simulink model "district_heating"  (R2018b)
settings: Solver=VariableStepAuto  StartTime=0.0  StopTime=24*3600  RelTol=1e-3
undefined symbols (not defined in the file): path_carnot
libraries: carnot x16, Pipe_BiFlow x2
settings Model: Creator=drhf  LastModifiedBy=drhf
settings SolverCC: AlgebraicLoopSolver=LineSearch

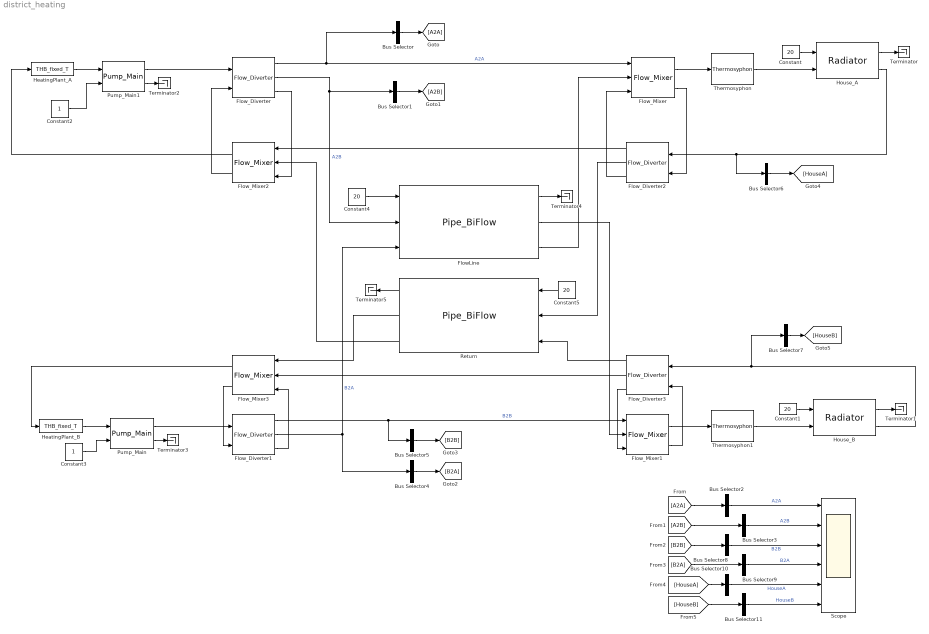
== system district_heating ==
  Bus Selector{,1,4..7} (6 alike) : BusSelector  OutputSignals=Temperature,MassFlow  OutputAsBus=on
  Bus Selector{2..3,8..11} (6 alike) : BusSelector  OutputSignals=MassFlow  OutputAsBus=on
  Constant{,1,4..5} (4 alike) : Constant  Value=20
  Constant2 : Constant
  Constant3 : Constant
  FlowLine : Pipe_BiFlow/Pipe_BiFlow  t0=20  hgt=254.6479  stgtype=1  tini=[20 20 20 20 20 20 20 20 20 20]  mpts=[1 2 3 4 5 6 7 8 9 10]  PathName=fullfile(path_carnot('libsl'),'Storage','Thermal','Storage_Type_1','parameter_set')  FileName='<user defined>'  userPath=off  userParam=on  uwall=1  ubot=1  utop=1  axcond=1  volume=2  dia=0.1  standing=standing cylinder  nodes=10  mpoints=10  pipe1inlet=1  pipe1outlet=0  pipe1dia=0.1  pipe2inlet=0  pipe2outlet=1  pipe2dia=0.1
  Flow_Diverter{,1..3} (4 alike) : carnot/Hydraulics/Flow_Diverter
      settings: SourceProductName=Carnot
  Flow_Mixer{,1..3} (4 alike) : carnot/Hydraulics/Flow_Mixer
      settings: SourceProductName=Carnot
  HeatingPlant_A : carnot/Source/Simple/THB_fixed_T  t=70
      settings: SourceProductName=Carnot
  HeatingPlant_B : carnot/Source/Simple/THB_fixed_T  t=60
      settings: SourceProductName=Carnot
  House_A : carnot/Source/Heat_Exchanger/Radiator  pnom=500  dtnom=49.83  expo=1.3  mcap=5*4182  tini=20  lin=10  qua=10
      settings: SourceProductName=Carnot
  House_B : carnot/Source/Heat_Exchanger/Radiator  pnom=500  dtnom=49.83  expo=1.3  mcap=5*4182  tini=20  lin=10  qua=10
      settings: SourceProductName=Carnot
  Pump_Main : carnot/Hydraulics/Pump_Main  Tini=20  p0=3e5  IDpreset=pressure drop  fluid=Water  mix=0  mix2=0  mix3=0  t1=1  PathName=fullfile(path_carnot('libsl'), 'Hydraulics', 'Pump_Main', 'parameter_set')  FileName='Pump6m.mat'  userPath=off  userParam=off  a0=60000  a1=-43200  a2=0  dia=0.025  UA=1  mcp=4182  e0=50  e1=28.8  e2=-10.368
      settings: SourceProductName=Carnot
  Pump_Main1 : carnot/Hydraulics/Pump_Main  Tini=20  p0=3e5  IDpreset=pressure drop  fluid=Water  mix=0  mix2=0  mix3=0  t1=1  PathName=fullfile(path_carnot('libsl'), 'Hydraulics', 'Pump_Main', 'parameter_set')  FileName='Pump8m.mat'  userPath=off  userParam=off  a0=80000  a1=-32000  a2=0  dia=0.025  UA=1  mcp=4182  e0=100  e1=36  e2=-6.4
      settings: SourceProductName=Carnot
  Return : Pipe_BiFlow/Pipe_BiFlow  t0=20  hgt=254.6479  stgtype=1  tini=[20 20 20 20 20 20 20 20 20 20]  mpts=[1 2 3 4 5 6 7 8 9 10]  PathName=fullfile(path_carnot('libsl'),'Storage','Thermal','Storage_Type_1','parameter_set')  FileName='<user defined>'  userPath=off  userParam=on  uwall=1  ubot=1  utop=1  axcond=1  volume=2  dia=0.1  standing=standing cylinder  nodes=10  mpoints=10  pipe1inlet=1  pipe1outlet=0  pipe1dia=0.1  pipe2inlet=0  pipe2outlet=1  pipe2dia=0.1
  Scope : Scope  NumInputPorts=6
  Terminator{,1..5} (6 alike) : Terminator
  Thermosyphon : carnot/Hydraulics/Thermosyphon  p0=3e5  dia=0.025  fluid_id=Water  mix=0  mix2=0  mix3=0  t1=1
      settings: SourceProductName=Carnot
  Thermosyphon1 : carnot/Hydraulics/Thermosyphon  p0=3e5  dia=0.025  fluid_id=Water  mix=0  mix2=0  mix3=0  t1=1
      settings: SourceProductName=Carnot
  wires:
  Constant/1 -> House_A/1
  House_A/1 -> Terminator/1
  HeatingPlant_B/1 -> Pump_Main/1
  HeatingPlant_A/1 -> Pump_Main1/1
  House_B/1 -> Terminator1/1
  Constant1/1 -> House_B/1
  Pump_Main1/2 -> Terminator2/1
  Pump_Main/2 -> Terminator3/1
  Constant2/1 -> Pump_Main1/2
  Constant3/1 -> Pump_Main/2
  Constant4/1 -> FlowLine/1
  Pump_Main1/1 -> Flow_Diverter/1
  Pump_Main/1 -> Flow_Diverter1/1
  FlowLine/1 -> Terminator4/1
  Constant5/1 -> Return/1
  Flow_Diverter/1 -> Flow_Mixer/1, Bus Selector/1  "A2A"
  Flow_Mixer/1 -> Thermosyphon/1
  FlowLine/3 -> Flow_Mixer/2
  Flow_Mixer1/1 -> Thermosyphon1/1
  FlowLine/2 -> Flow_Mixer1/2
  Flow_Diverter1/1 -> Bus Selector5/1, Flow_Mixer1/1  "B2B"
  House_A/2 -> Bus Selector6/1, Flow_Diverter2/1
  Flow_Diverter2/1 -> Flow_Mixer2/1
  Flow_Diverter2/2 -> Return/2
  Flow_Mixer2/1 -> HeatingPlant_A/1
  Return/2 -> Flow_Mixer3/1
  Flow_Mixer3/1 -> HeatingPlant_B/1
  House_B/2 -> Flow_Diverter3/1, Bus Selector7/1
  Flow_Diverter3/1 -> Return/3
  Flow_Diverter3/2 -> Flow_Mixer3/2
  Return/3 -> Flow_Mixer2/2
  Return/1 -> Terminator5/1
  Flow_Diverter2/3 -> Flow_Mixer/3
  Flow_Mixer/2 -> Flow_Diverter2/2
  Flow_Mixer1/2 -> Flow_Diverter3/2
  Flow_Diverter3/3 -> Flow_Mixer1/3
  Flow_Diverter1/3 -> Flow_Mixer3/3
  Flow_Mixer3/2 -> Flow_Diverter1/2
  Flow_Mixer2/2 -> Flow_Diverter/2
  Flow_Diverter/3 -> Flow_Mixer2/3
  Thermosyphon/1 -> House_A/2
  Thermosyphon1/1 -> House_B/2
  Bus Selector/1 -> [A2A]
  Bus Selector1/1 -> [A2B]
  Flow_Diverter/2 -> FlowLine/2, Bus Selector1/1  "A2B"
  [A2A] -> Bus Selector2/1
  Bus Selector2/1 -> Scope/1  "A2A"
  [A2B] -> Bus Selector3/1
  Bus Selector3/1 -> Scope/2  "A2B"
  Flow_Diverter1/2 -> Bus Selector4/1, FlowLine/3  "B2A"
  Bus Selector4/1 -> [B2A]
  Bus Selector5/1 -> [B2B]
  Bus Selector6/1 -> [HouseA]
  Bus Selector7/1 -> [HouseB]
  [B2B] -> Bus Selector8/1
  [B2A] -> Bus Selector9/1
  [HouseA] -> Bus Selector10/1
  [HouseB] -> Bus Selector11/1
  Bus Selector8/1 -> Scope/3  "B2B"
  Bus Selector9/1 -> Scope/4  "B2A"
  Bus Selector10/1 -> Scope/5  "HouseA"
  Bus Selector11/1 -> Scope/6  "HouseB"
